simulink model "Status_Checking"  (R2023b)
settings: Solver=VariableStepAuto  StartTime=0.0  StopTime=10.0  RelTol=1e-3
settings Model: Creator=pmodi  LastModifiedBy=pmodi

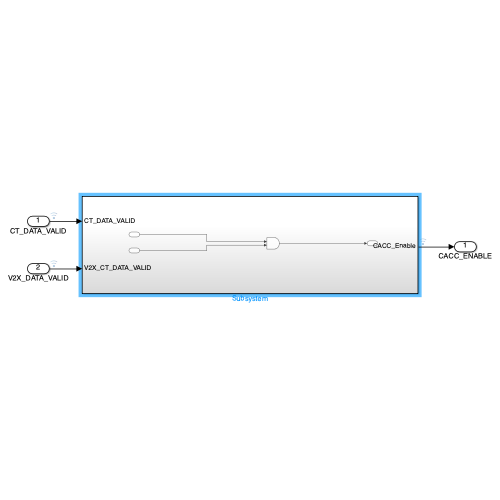
[thumbnail: Simulink's stored preview of the top-level diagram]
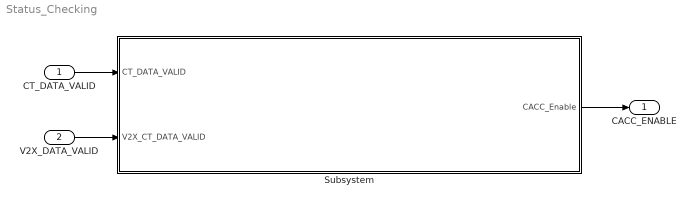
== system Status_Checking ==
  CT_DATA_VALID : Inport
  V2X_DATA_VALID : Inport  Port=2
  Subsystem : Subsystem
  CACC_ENABLE : Outport
  wires:
  CT_DATA_VALID/1 -> Subsystem/1(CT_DATA_VALID)
  V2X_DATA_VALID/1 -> Subsystem/2(V2X_CT_DATA_VALID)
  Subsystem/1(CACC_Enable) -> CACC_ENABLE/1

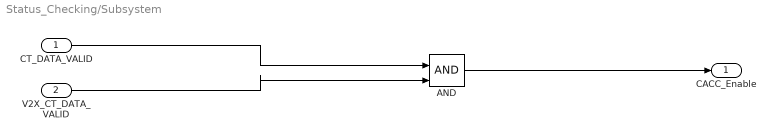
== system Status_Checking/Subsystem ==
  CT_DATA_VALID : Inport
  V2X_CT_DATA_VALID : Inport  Port=2
  AND : Logic  IconShape=distinctive  AllPortsSameDT=off  OutDataTypeStr=boolean
  CACC_Enable : Outport  VectorParamsAs1DForOutWhenUnconnected=off
  wires:
  CT_DATA_VALID/1 -> AND/1
  V2X_CT_DATA_VALID/1 -> AND/2
  AND/1 -> CACC_Enable/1
